simulink model "twoOctave"  (R2015a)
settings: Solver=ode45  StartTime=0.0  StopTime=480*640+7000  RelTol=1e-3
InitFcn:
  | %% DSPBuilder Start
  | alt_dspbuilder_update_model(bdroot)
  | %% DSPBuilder End
libraries: allblocks_alteradspbuilder2 x1298
(part 2 of 16)

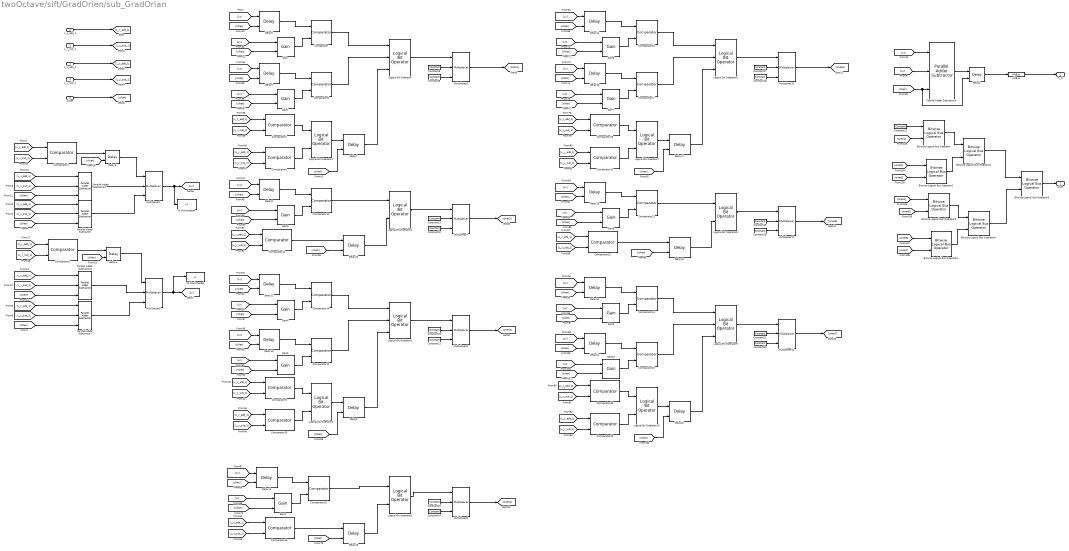
== system twoOctave/sift/GradOrien/sub_GradOrian ==
  L_y_add_1 : Inport
  L_x_add_1 : Inport  Port=2
  L_x_sub_1 : Inport  Port=3
  L_y_sub_1 : Inport  Port=4
  clken : Inport  Port=5
  AltBus : allblocks_alteradspbuilder2/AltBus  BusType=Unsigned Fractional  bwl=10  bwr=16  saturate=off  floatingPointInput=on  floatingPointOutput=on  logOutputs=off  logFile=C:\Users\ASUS\Desktop\final_sift_fpga\tb_twoOctave\twoOctave_sift_GradOrien_sub%5FGradOrian_AltBus.fixedpointlog
  Bitwise Logical Bus Operator{,1..6} (7 alike) : allblocks_alteradspbuilder2/Bitwise Logical Bus Operator  BusType=Unsigned Integer  bwl=3  bwr=0  LogicalOperator=OR  pipeline_display=0
  Comparator : allblocks_alteradspbuilder2/Comparator  direction=a >= b  pipeline_display=0  allowFloatingPointOverride=on  logOutputs=off  logFile=C:\Users\ASUS\Desktop\final_sift_fpga\tb_twoOctave\twoOctave_sift_GradOrien_sub%5FGradOrian_Comparator.fixedpointlog
  Comparator1 : allblocks_alteradspbuilder2/Comparator  direction=a > b  pipeline_display=0  allowFloatingPointOverride=on  logOutputs=off  logFile=C:\Users\ASUS\Desktop\final_sift_fpga\tb_twoOctave\twoOctave_sift_GradOrien_sub%5FGradOrian_Comparator1.fixedpointlog
  Comparator10 : allblocks_alteradspbuilder2/Comparator  direction=a >= b  pipeline_display=0  allowFloatingPointOverride=on  logOutputs=off  logFile=C:\Users\ASUS\Desktop\final_sift_fpga\tb_twoOctave\twoOctave_sift_GradOrien_sub%5FGradOrian_Comparator10.fixedpointlog
  Comparator11 : allblocks_alteradspbuilder2/Comparator  direction=a < b  pipeline_display=0  allowFloatingPointOverride=on  logOutputs=off  logFile=C:\Users\ASUS\Desktop\final_sift_fpga\tb_twoOctave\twoOctave_sift_GradOrien_sub%5FGradOrian_Comparator11.fixedpointlog
  Comparator12 : allblocks_alteradspbuilder2/Comparator  direction=a > b  pipeline_display=0  allowFloatingPointOverride=on  logOutputs=off  logFile=C:\Users\ASUS\Desktop\final_sift_fpga\tb_twoOctave\twoOctave_sift_GradOrien_sub%5FGradOrian_Comparator12.fixedpointlog
  Comparator13 : allblocks_alteradspbuilder2/Comparator  direction=a >= b  pipeline_display=0  allowFloatingPointOverride=on  logOutputs=off  logFile=C:\Users\ASUS\Desktop\final_sift_fpga\tb_twoOctave\twoOctave_sift_GradOrien_sub%5FGradOrian_Comparator13.fixedpointlog
  Comparator14 : allblocks_alteradspbuilder2/Comparator  direction=a >= b  pipeline_display=0  allowFloatingPointOverride=on  logOutputs=off  logFile=C:\Users\ASUS\Desktop\final_sift_fpga\tb_twoOctave\twoOctave_sift_GradOrien_sub%5FGradOrian_Comparator14.fixedpointlog
  Comparator15 : allblocks_alteradspbuilder2/Comparator  direction=a > b  pipeline_display=0  allowFloatingPointOverride=on  logOutputs=off  logFile=C:\Users\ASUS\Desktop\final_sift_fpga\tb_twoOctave\twoOctave_sift_GradOrien_sub%5FGradOrian_Comparator15.fixedpointlog
  Comparator16 : allblocks_alteradspbuilder2/Comparator  direction=a < b  pipeline_display=0  allowFloatingPointOverride=on  logOutputs=off  logFile=C:\Users\ASUS\Desktop\final_sift_fpga\tb_twoOctave\twoOctave_sift_GradOrien_sub%5FGradOrian_Comparator16.fixedpointlog
  Comparator17 : allblocks_alteradspbuilder2/Comparator  direction=a < b  pipeline_display=0  allowFloatingPointOverride=on  logOutputs=off  logFile=C:\Users\ASUS\Desktop\final_sift_fpga\tb_twoOctave\twoOctave_sift_GradOrien_sub%5FGradOrian_Comparator17.fixedpointlog
  Comparator18 : allblocks_alteradspbuilder2/Comparator  direction=a < b  pipeline_display=0  allowFloatingPointOverride=on  logOutputs=off  logFile=C:\Users\ASUS\Desktop\final_sift_fpga\tb_twoOctave\twoOctave_sift_GradOrien_sub%5FGradOrian_Comparator18.fixedpointlog
  Comparator19 : allblocks_alteradspbuilder2/Comparator  direction=a < b  pipeline_display=0  allowFloatingPointOverride=on  logOutputs=off  logFile=C:\Users\ASUS\Desktop\final_sift_fpga\tb_twoOctave\twoOctave_sift_GradOrien_sub%5FGradOrian_Comparator19.fixedpointlog
  Comparator2 : allblocks_alteradspbuilder2/Comparator  direction=a > b  pipeline_display=0  allowFloatingPointOverride=on  logOutputs=off  logFile=C:\Users\ASUS\Desktop\final_sift_fpga\tb_twoOctave\twoOctave_sift_GradOrien_sub%5FGradOrian_Comparator2.fixedpointlog
  Comparator20 : allblocks_alteradspbuilder2/Comparator  direction=a < b  pipeline_display=0  allowFloatingPointOverride=on  logOutputs=off  logFile=C:\Users\ASUS\Desktop\final_sift_fpga\tb_twoOctave\twoOctave_sift_GradOrien_sub%5FGradOrian_Comparator20.fixedpointlog
  Comparator21 : allblocks_alteradspbuilder2/Comparator  direction=a >= b  pipeline_display=0  allowFloatingPointOverride=on  logOutputs=off  logFile=C:\Users\ASUS\Desktop\final_sift_fpga\tb_twoOctave\twoOctave_sift_GradOrien_sub%5FGradOrian_Comparator21.fixedpointlog
  Comparator22 : allblocks_alteradspbuilder2/Comparator  direction=a < b  pipeline_display=0  allowFloatingPointOverride=on  logOutputs=off  logFile=C:\Users\ASUS\Desktop\final_sift_fpga\tb_twoOctave\twoOctave_sift_GradOrien_sub%5FGradOrian_Comparator22.fixedpointlog
  Comparator23 : allblocks_alteradspbuilder2/Comparator  direction=a < b  pipeline_display=0  allowFloatingPointOverride=on  logOutputs=off  logFile=C:\Users\ASUS\Desktop\final_sift_fpga\tb_twoOctave\twoOctave_sift_GradOrien_sub%5FGradOrian_Comparator23.fixedpointlog
  Comparator24 : allblocks_alteradspbuilder2/Comparator  direction=a >= b  pipeline_display=0  allowFloatingPointOverride=on  logOutputs=off  logFile=C:\Users\ASUS\Desktop\final_sift_fpga\tb_twoOctave\twoOctave_sift_GradOrien_sub%5FGradOrian_Comparator24.fixedpointlog
  Comparator25 : allblocks_alteradspbuilder2/Comparator  direction=a < b  pipeline_display=0  allowFloatingPointOverride=on  logOutputs=off  logFile=C:\Users\ASUS\Desktop\final_sift_fpga\tb_twoOctave\twoOctave_sift_GradOrien_sub%5FGradOrian_Comparator25.fixedpointlog
  Comparator26 : allblocks_alteradspbuilder2/Comparator  direction=a > b  pipeline_display=0  allowFloatingPointOverride=on  logOutputs=off  logFile=C:\Users\ASUS\Desktop\final_sift_fpga\tb_twoOctave\twoOctave_sift_GradOrien_sub%5FGradOrian_Comparator26.fixedpointlog
  Comparator6 : allblocks_alteradspbuilder2/Comparator  direction=a < b  pipeline_display=0  allowFloatingPointOverride=on  logOutputs=off  logFile=C:\Users\ASUS\Desktop\final_sift_fpga\tb_twoOctave\twoOctave_sift_GradOrien_sub%5FGradOrian_Comparator6.fixedpointlog
  Comparator7 : allblocks_alteradspbuilder2/Comparator  direction=a > b  pipeline_display=0  allowFloatingPointOverride=on  logOutputs=off  logFile=C:\Users\ASUS\Desktop\final_sift_fpga\tb_twoOctave\twoOctave_sift_GradOrien_sub%5FGradOrian_Comparator7.fixedpointlog
  Comparator8 : allblocks_alteradspbuilder2/Comparator  direction=a > b  pipeline_display=0  allowFloatingPointOverride=on  logOutputs=off  logFile=C:\Users\ASUS\Desktop\final_sift_fpga\tb_twoOctave\twoOctave_sift_GradOrien_sub%5FGradOrian_Comparator8.fixedpointlog
  Comparator9 : allblocks_alteradspbuilder2/Comparator  direction=a < b  pipeline_display=0  allowFloatingPointOverride=on  logOutputs=off  logFile=C:\Users\ASUS\Desktop\final_sift_fpga\tb_twoOctave\twoOctave_sift_GradOrien_sub%5FGradOrian_Comparator9.fixedpointlog
  Constant10 : allblocks_alteradspbuilder2/Constant  mask_cst=2  BusType=Unsigned Integer  bwl=3  bwr=0  roundMode=Truncate  satMode=Wrap  SpecifyClock=off  allowFloatingPointOverride=on  logOutputs=off  logFile=C:\Users\ASUS\Desktop\final_sift_fpga\tb_twoOctave\twoOctave_sift_GradOrien_sub%5FGradOrian_Constant10.fixedpointlog
  Constant11 : allblocks_alteradspbuilder2/Constant  mask_cst=0  BusType=Unsigned Integer  bwl=3  bwr=0  roundMode=Truncate  satMode=Wrap  SpecifyClock=off  allowFloatingPointOverride=on  logOutputs=off  logFile=C:\Users\ASUS\Desktop\final_sift_fpga\tb_twoOctave\twoOctave_sift_GradOrien_sub%5FGradOrian_Constant11.fixedpointlog
  Constant12 : allblocks_alteradspbuilder2/Constant  mask_cst=3  BusType=Unsigned Integer  bwl=3  bwr=0  roundMode=Truncate  satMode=Wrap  SpecifyClock=off  allowFloatingPointOverride=on  logOutputs=off  logFile=C:\Users\ASUS\Desktop\final_sift_fpga\tb_twoOctave\twoOctave_sift_GradOrien_sub%5FGradOrian_Constant12.fixedpointlog
  Constant13 : allblocks_alteradspbuilder2/Constant  mask_cst=0  BusType=Unsigned Integer  bwl=3  bwr=0  roundMode=Truncate  satMode=Wrap  SpecifyClock=off  allowFloatingPointOverride=on  logOutputs=off  logFile=C:\Users\ASUS\Desktop\final_sift_fpga\tb_twoOctave\twoOctave_sift_GradOrien_sub%5FGradOrian_Constant13.fixedpointlog
  Constant14 : allblocks_alteradspbuilder2/Constant  mask_cst=4  BusType=Unsigned Integer  bwl=3  bwr=0  roundMode=Truncate  satMode=Wrap  SpecifyClock=off  allowFloatingPointOverride=on  logOutputs=off  logFile=C:\Users\ASUS\Desktop\final_sift_fpga\tb_twoOctave\twoOctave_sift_GradOrien_sub%5FGradOrian_Constant14.fixedpointlog
  Constant15 : allblocks_alteradspbuilder2/Constant  mask_cst=0  BusType=Unsigned Integer  bwl=3  bwr=0  roundMode=Truncate  satMode=Wrap  SpecifyClock=off  allowFloatingPointOverride=on  logOutputs=off  logFile=C:\Users\ASUS\Desktop\final_sift_fpga\tb_twoOctave\twoOctave_sift_GradOrien_sub%5FGradOrian_Constant15.fixedpointlog
  Constant16 : allblocks_alteradspbuilder2/Constant  mask_cst=5  BusType=Unsigned Integer  bwl=3  bwr=0  roundMode=Truncate  satMode=Wrap  SpecifyClock=off  allowFloatingPointOverride=on  logOutputs=off  logFile=C:\Users\ASUS\Desktop\final_sift_fpga\tb_twoOctave\twoOctave_sift_GradOrien_sub%5FGradOrian_Constant16.fixedpointlog
  Constant17 : allblocks_alteradspbuilder2/Constant  mask_cst=0  BusType=Unsigned Integer  bwl=3  bwr=0  roundMode=Truncate  satMode=Wrap  SpecifyClock=off  allowFloatingPointOverride=on  logOutputs=off  logFile=C:\Users\ASUS\Desktop\final_sift_fpga\tb_twoOctave\twoOctave_sift_GradOrien_sub%5FGradOrian_Constant17.fixedpointlog
  Constant18 : allblocks_alteradspbuilder2/Constant  mask_cst=6  BusType=Unsigned Integer  bwl=3  bwr=0  roundMode=Truncate  satMode=Wrap  SpecifyClock=off  allowFloatingPointOverride=on  logOutputs=off  logFile=C:\Users\ASUS\Desktop\final_sift_fpga\tb_twoOctave\twoOctave_sift_GradOrien_sub%5FGradOrian_Constant18.fixedpointlog
  Constant19 : allblocks_alteradspbuilder2/Constant  mask_cst=0  BusType=Unsigned Integer  bwl=3  bwr=0  roundMode=Truncate  satMode=Wrap  SpecifyClock=off  allowFloatingPointOverride=on  logOutputs=off  logFile=C:\Users\ASUS\Desktop\final_sift_fpga\tb_twoOctave\twoOctave_sift_GradOrien_sub%5FGradOrian_Constant19.fixedpointlog
  Constant20 : allblocks_alteradspbuilder2/Constant  mask_cst=7  BusType=Unsigned Integer  bwl=3  bwr=0  roundMode=Truncate  satMode=Wrap  SpecifyClock=off  allowFloatingPointOverride=on  logOutputs=off  logFile=C:\Users\ASUS\Desktop\final_sift_fpga\tb_twoOctave\twoOctave_sift_GradOrien_sub%5FGradOrian_Constant20.fixedpointlog
  Constant21 : allblocks_alteradspbuilder2/Constant  mask_cst=0  BusType=Unsigned Integer  bwl=3  bwr=0  roundMode=Truncate  satMode=Wrap  SpecifyClock=off  allowFloatingPointOverride=on  logOutputs=off  logFile=C:\Users\ASUS\Desktop\final_sift_fpga\tb_twoOctave\twoOctave_sift_GradOrien_sub%5FGradOrian_Constant21.fixedpointlog
  Constant22 : allblocks_alteradspbuilder2/Constant  mask_cst=0  BusType=Unsigned Integer  bwl=3  bwr=0  roundMode=Truncate  satMode=Wrap  SpecifyClock=off  allowFloatingPointOverride=on  logOutputs=off  logFile=C:\Users\ASUS\Desktop\final_sift_fpga\tb_twoOctave\twoOctave_sift_GradOrien_sub%5FGradOrian_Constant22.fixedpointlog
  Constant8 : allblocks_alteradspbuilder2/Constant  mask_cst=1  BusType=Unsigned Integer  bwl=3  bwr=0  roundMode=Truncate  satMode=Wrap  SpecifyClock=off  allowFloatingPointOverride=on  logOutputs=off  logFile=C:\Users\ASUS\Desktop\final_sift_fpga\tb_twoOctave\twoOctave_sift_GradOrien_sub%5FGradOrian_Constant8.fixedpointlog
  Constant9 : allblocks_alteradspbuilder2/Constant  mask_cst=0  BusType=Unsigned Integer  bwl=3  bwr=0  roundMode=Truncate  satMode=Wrap  SpecifyClock=off  allowFloatingPointOverride=on  logOutputs=off  logFile=C:\Users\ASUS\Desktop\final_sift_fpga\tb_twoOctave\twoOctave_sift_GradOrien_sub%5FGradOrian_Constant9.fixedpointlog
  Delay1 : allblocks_alteradspbuilder2/Delay  pipeline=15  pipeline_display=15  ClockPhase=1  use_ena=on  use_sclr=off  allowFloatingPointOverride=on  logOutputs=off  logFile=C:\Users\ASUS\Desktop\final_sift_fpga\tb_twoOctave\twoOctave_sift_GradOrien_sub%5FGradOrian_Delay1.fixedpointlog  use_init=off  reset_value=1
  Delay10 : allblocks_alteradspbuilder2/Delay  pipeline=17  pipeline_display=17  ClockPhase=1  use_ena=on  use_sclr=off  allowFloatingPointOverride=on  logOutputs=off  logFile=C:\Users\ASUS\Desktop\final_sift_fpga\tb_twoOctave\twoOctave_sift_GradOrien_sub%5FGradOrian_Delay10.fixedpointlog  use_init=off  reset_value=1
  Delay11 : allblocks_alteradspbuilder2/Delay  pipeline=16  pipeline_display=16  ClockPhase=1  use_ena=on  use_sclr=off  allowFloatingPointOverride=on  logOutputs=off  logFile=C:\Users\ASUS\Desktop\final_sift_fpga\tb_twoOctave\twoOctave_sift_GradOrien_sub%5FGradOrian_Delay11.fixedpointlog  use_init=off  reset_value=1
  Delay12 : allblocks_alteradspbuilder2/Delay  pipeline=16  pipeline_display=16  ClockPhase=1  use_ena=on  use_sclr=off  allowFloatingPointOverride=on  logOutputs=off  logFile=C:\Users\ASUS\Desktop\final_sift_fpga\tb_twoOctave\twoOctave_sift_GradOrien_sub%5FGradOrian_Delay12.fixedpointlog  use_init=off  reset_value=1
  Delay13 : allblocks_alteradspbuilder2/Delay  pipeline=16  pipeline_display=16  ClockPhase=1  use_ena=on  use_sclr=off  allowFloatingPointOverride=on  logOutputs=off  logFile=C:\Users\ASUS\Desktop\final_sift_fpga\tb_twoOctave\twoOctave_sift_GradOrien_sub%5FGradOrian_Delay13.fixedpointlog  use_init=off  reset_value=1
  Delay14 : allblocks_alteradspbuilder2/Delay  pipeline=16  pipeline_display=16  ClockPhase=1  use_ena=on  use_sclr=off  allowFloatingPointOverride=on  logOutputs=off  logFile=C:\Users\ASUS\Desktop\final_sift_fpga\tb_twoOctave\twoOctave_sift_GradOrien_sub%5FGradOrian_Delay14.fixedpointlog  use_init=off  reset_value=1
  Delay15 : allblocks_alteradspbuilder2/Delay  pipeline=17  pipeline_display=17  ClockPhase=1  use_ena=on  use_sclr=off  allowFloatingPointOverride=on  logOutputs=off  logFile=C:\Users\ASUS\Desktop\final_sift_fpga\tb_twoOctave\twoOctave_sift_GradOrien_sub%5FGradOrian_Delay15.fixedpointlog  use_init=off  reset_value=1
  Delay16 : allblocks_alteradspbuilder2/Delay  pipeline=16  pipeline_display=16  ClockPhase=1  use_ena=on  use_sclr=off  allowFloatingPointOverride=on  logOutputs=off  logFile=C:\Users\ASUS\Desktop\final_sift_fpga\tb_twoOctave\twoOctave_sift_GradOrien_sub%5FGradOrian_Delay16.fixedpointlog  use_init=off  reset_value=1
  Delay17 : allblocks_alteradspbuilder2/Delay  pipeline=17  pipeline_display=17  ClockPhase=1  use_ena=on  use_sclr=off  allowFloatingPointOverride=on  logOutputs=off  logFile=C:\Users\ASUS\Desktop\final_sift_fpga\tb_twoOctave\twoOctave_sift_GradOrien_sub%5FGradOrian_Delay17.fixedpointlog  use_init=off  reset_value=1
  Delay18 : allblocks_alteradspbuilder2/Delay  pipeline=17  pipeline_display=17  ClockPhase=1  use_ena=on  use_sclr=off  allowFloatingPointOverride=on  logOutputs=off  logFile=C:\Users\ASUS\Desktop\final_sift_fpga\tb_twoOctave\twoOctave_sift_GradOrien_sub%5FGradOrian_Delay18.fixedpointlog  use_init=off  reset_value=1
  Delay19 : allblocks_alteradspbuilder2/Delay  pipeline=16  pipeline_display=16  ClockPhase=1  use_ena=on  use_sclr=off  allowFloatingPointOverride=on  logOutputs=off  logFile=C:\Users\ASUS\Desktop\final_sift_fpga\tb_twoOctave\twoOctave_sift_GradOrien_sub%5FGradOrian_Delay19.fixedpointlog  use_init=off  reset_value=1
  Delay20 : allblocks_alteradspbuilder2/Delay  pipeline=16  pipeline_display=16  ClockPhase=1  use_ena=on  use_sclr=off  allowFloatingPointOverride=on  logOutputs=off  logFile=C:\Users\ASUS\Desktop\final_sift_fpga\tb_twoOctave\twoOctave_sift_GradOrien_sub%5FGradOrian_Delay20.fixedpointlog  use_init=off  reset_value=1
  Delay21 : allblocks_alteradspbuilder2/Delay  pipeline=16  pipeline_display=16  ClockPhase=1  use_ena=on  use_sclr=off  allowFloatingPointOverride=on  logOutputs=off  logFile=C:\Users\ASUS\Desktop\final_sift_fpga\tb_twoOctave\twoOctave_sift_GradOrien_sub%5FGradOrian_Delay21.fixedpointlog  use_init=off  reset_value=1
  Delay22 : allblocks_alteradspbuilder2/Delay  pipeline=17  pipeline_display=17  ClockPhase=1  use_ena=on  use_sclr=off  allowFloatingPointOverride=on  logOutputs=off  logFile=C:\Users\ASUS\Desktop\final_sift_fpga\tb_twoOctave\twoOctave_sift_GradOrien_sub%5FGradOrian_Delay22.fixedpointlog  use_init=off  reset_value=1
  Delay3 : allblocks_alteradspbuilder2/Delay  pipeline=1  pipeline_display=1  ClockPhase=1  use_ena=on  use_sclr=off  allowFloatingPointOverride=on  logOutputs=off  logFile=C:\Users\ASUS\Desktop\final_sift_fpga\tb_twoOctave\twoOctave_sift_GradOrien_sub%5FGradOrian_Delay3.fixedpointlog  use_init=off  reset_value=1
  Delay4 : allblocks_alteradspbuilder2/Delay  pipeline=1  pipeline_display=1  ClockPhase=1  use_ena=on  use_sclr=off  allowFloatingPointOverride=on  logOutputs=off  logFile=C:\Users\ASUS\Desktop\final_sift_fpga\tb_twoOctave\twoOctave_sift_GradOrien_sub%5FGradOrian_Delay4.fixedpointlog  use_init=off  reset_value=1
  Delay5 : allblocks_alteradspbuilder2/Delay  pipeline=16  pipeline_display=16  ClockPhase=1  use_ena=on  use_sclr=off  allowFloatingPointOverride=on  logOutputs=off  logFile=C:\Users\ASUS\Desktop\final_sift_fpga\tb_twoOctave\twoOctave_sift_GradOrien_sub%5FGradOrian_Delay5.fixedpointlog  use_init=off  reset_value=1
  Delay6 : allblocks_alteradspbuilder2/Delay  pipeline=16  pipeline_display=16  ClockPhase=1  use_ena=on  use_sclr=off  allowFloatingPointOverride=on  logOutputs=off  logFile=C:\Users\ASUS\Desktop\final_sift_fpga\tb_twoOctave\twoOctave_sift_GradOrien_sub%5FGradOrian_Delay6.fixedpointlog  use_init=off  reset_value=1
  Delay7 : allblocks_alteradspbuilder2/Delay  pipeline=17  pipeline_display=17  ClockPhase=1  use_ena=on  use_sclr=off  allowFloatingPointOverride=on  logOutputs=off  logFile=C:\Users\ASUS\Desktop\final_sift_fpga\tb_twoOctave\twoOctave_sift_GradOrien_sub%5FGradOrian_Delay7.fixedpointlog  use_init=off  reset_value=1
  Delay8 : allblocks_alteradspbuilder2/Delay  pipeline=17  pipeline_display=17  ClockPhase=1  use_ena=on  use_sclr=off  allowFloatingPointOverride=on  logOutputs=off  logFile=C:\Users\ASUS\Desktop\final_sift_fpga\tb_twoOctave\twoOctave_sift_GradOrien_sub%5FGradOrian_Delay8.fixedpointlog  use_init=off  reset_value=1
  Delay9 : allblocks_alteradspbuilder2/Delay  pipeline=16  pipeline_display=16  ClockPhase=1  use_ena=on  use_sclr=off  allowFloatingPointOverride=on  logOutputs=off  logFile=C:\Users\ASUS\Desktop\final_sift_fpga\tb_twoOctave\twoOctave_sift_GradOrien_sub%5FGradOrian_Delay9.fixedpointlog  use_init=off  reset_value=1
  Gain : allblocks_alteradspbuilder2/Gain  vgain=0.414  BusType=Unsigned Fractional  bwl=8  bwr=16  pipeline=16  pipeline_display=16  allowFloatingPointOverride=on  logOutputs=off  logFile=C:\Users\ASUS\Desktop\final_sift_fpga\tb_twoOctave\twoOctave_sift_GradOrien_sub%5FGradOrian_Gain.fixedpointlog  use_ena=on  use_aclr=off  lpm=off  MaskValue=1
  Gain1 : allblocks_alteradspbuilder2/Gain  vgain=2.414  BusType=Unsigned Fractional  bwl=8  bwr=16  pipeline=16  pipeline_display=16  allowFloatingPointOverride=on  logOutputs=off  logFile=C:\Users\ASUS\Desktop\final_sift_fpga\tb_twoOctave\twoOctave_sift_GradOrien_sub%5FGradOrian_Gain1.fixedpointlog  use_ena=on  use_aclr=off  lpm=off  MaskValue=1
  Gain10 : allblocks_alteradspbuilder2/Gain  vgain=2.414  BusType=Unsigned Fractional  bwl=8  bwr=16  pipeline=16  pipeline_display=16  allowFloatingPointOverride=on  logOutputs=off  logFile=C:\Users\ASUS\Desktop\final_sift_fpga\tb_twoOctave\twoOctave_sift_GradOrien_sub%5FGradOrian_Gain10.fixedpointlog  use_ena=on  use_aclr=off  lpm=off  MaskValue=1
  Gain2 : allblocks_alteradspbuilder2/Gain  vgain=0.414  BusType=Unsigned Fractional  bwl=8  bwr=16  pipeline=16  pipeline_display=16  allowFloatingPointOverride=on  logOutputs=off  logFile=C:\Users\ASUS\Desktop\final_sift_fpga\tb_twoOctave\twoOctave_sift_GradOrien_sub%5FGradOrian_Gain2.fixedpointlog  use_ena=on  use_aclr=off  lpm=off  MaskValue=1
  Gain3 : allblocks_alteradspbuilder2/Gain  vgain=2.414  BusType=Unsigned Fractional  bwl=8  bwr=16  pipeline=16  pipeline_display=16  allowFloatingPointOverride=on  logOutputs=off  logFile=C:\Users\ASUS\Desktop\final_sift_fpga\tb_twoOctave\twoOctave_sift_GradOrien_sub%5FGradOrian_Gain3.fixedpointlog  use_ena=on  use_aclr=off  lpm=off  MaskValue=1
  Gain4 : allblocks_alteradspbuilder2/Gain  vgain=0.414  BusType=Unsigned Fractional  bwl=8  bwr=16  pipeline=16  pipeline_display=16  allowFloatingPointOverride=on  logOutputs=off  logFile=C:\Users\ASUS\Desktop\final_sift_fpga\tb_twoOctave\twoOctave_sift_GradOrien_sub%5FGradOrian_Gain4.fixedpointlog  use_ena=on  use_aclr=off  lpm=off  MaskValue=1
  Gain5 : allblocks_alteradspbuilder2/Gain  vgain=2.414  BusType=Unsigned Fractional  bwl=8  bwr=16  pipeline=16  pipeline_display=16  allowFloatingPointOverride=on  logOutputs=off  logFile=C:\Users\ASUS\Desktop\final_sift_fpga\tb_twoOctave\twoOctave_sift_GradOrien_sub%5FGradOrian_Gain5.fixedpointlog  use_ena=on  use_aclr=off  lpm=off  MaskValue=1
  Gain6 : allblocks_alteradspbuilder2/Gain  vgain=0.414  BusType=Unsigned Fractional  bwl=8  bwr=16  pipeline=16  pipeline_display=16  allowFloatingPointOverride=on  logOutputs=off  logFile=C:\Users\ASUS\Desktop\final_sift_fpga\tb_twoOctave\twoOctave_sift_GradOrien_sub%5FGradOrian_Gain6.fixedpointlog  use_ena=on  use_aclr=off  lpm=off  MaskValue=1
  Gain7 : allblocks_alteradspbuilder2/Gain  vgain=2.414  BusType=Unsigned Fractional  bwl=8  bwr=16  pipeline=16  pipeline_display=16  allowFloatingPointOverride=on  logOutputs=off  logFile=C:\Users\ASUS\Desktop\final_sift_fpga\tb_twoOctave\twoOctave_sift_GradOrien_sub%5FGradOrian_Gain7.fixedpointlog  use_ena=on  use_aclr=off  lpm=off  MaskValue=1
  Gain8 : allblocks_alteradspbuilder2/Gain  vgain=2.414  BusType=Unsigned Fractional  bwl=8  bwr=16  pipeline=16  pipeline_display=16  allowFloatingPointOverride=on  logOutputs=off  logFile=C:\Users\ASUS\Desktop\final_sift_fpga\tb_twoOctave\twoOctave_sift_GradOrien_sub%5FGradOrian_Gain8.fixedpointlog  use_ena=on  use_aclr=off  lpm=off  MaskValue=1
  Gain9 : allblocks_alteradspbuilder2/Gain  vgain=0.414  BusType=Unsigned Fractional  bwl=8  bwr=16  pipeline=16  pipeline_display=16  allowFloatingPointOverride=on  logOutputs=off  logFile=C:\Users\ASUS\Desktop\final_sift_fpga\tb_twoOctave\twoOctave_sift_GradOrien_sub%5FGradOrian_Gain9.fixedpointlog  use_ena=on  use_aclr=off  lpm=off  MaskValue=1
  Logical Bit Operator{,3,6,9} (4 alike) : allblocks_alteradspbuilder2/Logical Bit Operator  LogicalOperator=AND  user_inputs=3  pipeline_display=0
  Logical Bit Operator{1..2,4..5,7..8,10} (7 alike) : allblocks_alteradspbuilder2/Logical Bit Operator  LogicalOperator=AND  user_inputs=2  pipeline_display=0
  Multiplexer1 : allblocks_alteradspbuilder2/Multiplexer  numInputs=2  pipeline=0  oneHot=off  pipeline_display=0  use_ena=off  use_aclr=off  allowFloatingPointOverride=on  logOutputs=off  logFile=C:\Users\ASUS\Desktop\final_sift_fpga\tb_twoOctave\twoOctave_sift_GradOrien_sub%5FGradOrian_Multiplexer1.fixedpointlog
  Multiplexer10 : allblocks_alteradspbuilder2/Multiplexer  numInputs=2  pipeline=0  oneHot=off  pipeline_display=0  use_ena=off  use_aclr=off  allowFloatingPointOverride=on  logOutputs=off  logFile=C:\Users\ASUS\Desktop\final_sift_fpga\tb_twoOctave\twoOctave_sift_GradOrien_sub%5FGradOrian_Multiplexer10.fixedpointlog
  Multiplexer11 : allblocks_alteradspbuilder2/Multiplexer  numInputs=2  pipeline=0  oneHot=off  pipeline_display=0  use_ena=off  use_aclr=off  allowFloatingPointOverride=on  logOutputs=off  logFile=C:\Users\ASUS\Desktop\final_sift_fpga\tb_twoOctave\twoOctave_sift_GradOrien_sub%5FGradOrian_Multiplexer11.fixedpointlog
  Multiplexer12 : allblocks_alteradspbuilder2/Multiplexer  numInputs=2  pipeline=0  oneHot=off  pipeline_display=0  use_ena=off  use_aclr=off  allowFloatingPointOverride=on  logOutputs=off  logFile=C:\Users\ASUS\Desktop\final_sift_fpga\tb_twoOctave\twoOctave_sift_GradOrien_sub%5FGradOrian_Multiplexer12.fixedpointlog
  Multiplexer5 : allblocks_alteradspbuilder2/Multiplexer  numInputs=2  pipeline=0  oneHot=off  pipeline_display=0  use_ena=off  use_aclr=off  allowFloatingPointOverride=on  logOutputs=off  logFile=C:\Users\ASUS\Desktop\final_sift_fpga\tb_twoOctave\twoOctave_sift_GradOrien_sub%5FGradOrian_Multiplexer5.fixedpointlog
  Multiplexer6 : allblocks_alteradspbuilder2/Multiplexer  numInputs=2  pipeline=0  oneHot=off  pipeline_display=0  use_ena=off  use_aclr=off  allowFloatingPointOverride=on  logOutputs=off  logFile=C:\Users\ASUS\Desktop\final_sift_fpga\tb_twoOctave\twoOctave_sift_GradOrien_sub%5FGradOrian_Multiplexer6.fixedpointlog
  Multiplexer7 : allblocks_alteradspbuilder2/Multiplexer  numInputs=2  pipeline=0  oneHot=off  pipeline_display=0  use_ena=off  use_aclr=off  allowFloatingPointOverride=on  logOutputs=off  logFile=C:\Users\ASUS\Desktop\final_sift_fpga\tb_twoOctave\twoOctave_sift_GradOrien_sub%5FGradOrian_Multiplexer7.fixedpointlog
  Multiplexer8 : allblocks_alteradspbuilder2/Multiplexer  numInputs=2  pipeline=0  oneHot=off  pipeline_display=0  use_ena=off  use_aclr=off  allowFloatingPointOverride=on  logOutputs=off  logFile=C:\Users\ASUS\Desktop\final_sift_fpga\tb_twoOctave\twoOctave_sift_GradOrien_sub%5FGradOrian_Multiplexer8.fixedpointlog
  Multiplexer9 : allblocks_alteradspbuilder2/Multiplexer  numInputs=2  pipeline=0  oneHot=off  pipeline_display=0  use_ena=off  use_aclr=off  allowFloatingPointOverride=on  logOutputs=off  logFile=C:\Users\ASUS\Desktop\final_sift_fpga\tb_twoOctave\twoOctave_sift_GradOrien_sub%5FGradOrian_Multiplexer9.fixedpointlog
  Parallel Adder Subtractor : allblocks_alteradspbuilder2/Parallel Adder Subtractor  number_of_inputs=2  direction=+-  use_pipeline=on  pipeline_display=1  phase_selection=1  use_ena=on  use_aclr=off  allowFloatingPointOverride=on  logOutputs=off  logFile=C:\Users\ASUS\Desktop\final_sift_fpga\tb_twoOctave\twoOctave_sift_GradOrien_sub%5FGradOrian_Parallel+Adder+Subtractor.fixedpointlog
  Parallel Adder Subtractor1 : allblocks_alteradspbuilder2/Parallel Adder Subtractor  number_of_inputs=2  direction=+-  use_pipeline=on  pipeline_display=1  phase_selection=1  use_ena=on  use_aclr=off  allowFloatingPointOverride=on  logOutputs=off  logFile=C:\Users\ASUS\Desktop\final_sift_fpga\tb_twoOctave\twoOctave_sift_GradOrien_sub%5FGradOrian_Parallel+Adder+Subtractor1.fixedpointlog
  Parallel Adder Subtractor2 : allblocks_alteradspbuilder2/Parallel Adder Subtractor  number_of_inputs=2  direction=-+  use_pipeline=on  pipeline_display=1  phase_selection=1  use_ena=on  use_aclr=off  allowFloatingPointOverride=on  logOutputs=off  logFile=C:\Users\ASUS\Desktop\final_sift_fpga\tb_twoOctave\twoOctave_sift_GradOrien_sub%5FGradOrian_Parallel+Adder+Subtractor2.fixedpointlog
  Parallel Adder Subtractor3 : allblocks_alteradspbuilder2/Parallel Adder Subtractor  number_of_inputs=2  direction=-+  use_pipeline=on  pipeline_display=1  phase_selection=1  use_ena=on  use_aclr=off  allowFloatingPointOverride=on  logOutputs=off  logFile=C:\Users\ASUS\Desktop\final_sift_fpga\tb_twoOctave\twoOctave_sift_GradOrien_sub%5FGradOrian_Parallel+Adder+Subtractor3.fixedpointlog
  Parallel Adder Subtractor5 : allblocks_alteradspbuilder2/Parallel Adder Subtractor  number_of_inputs=2  direction=++  use_pipeline=on  pipeline_display=1  phase_selection=1  use_ena=on  use_aclr=off  allowFloatingPointOverride=on  logOutputs=off  logFile=C:\Users\ASUS\Desktop\final_sift_fpga\tb_twoOctave\twoOctave_sift_GradOrien_sub%5FGradOrian_Parallel+Adder+Subtractor5.fixedpointlog
  To Workspace4 : ToWorkspace  VariableName=Lx  SaveFormat=Timeseries  SampleTime=-1
  To Workspace6 : ToWorkspace  VariableName=Ly  SaveFormat=Timeseries  SampleTime=-1
  orien : Outport
  m_xy : Outport  Port=2
  wires:
  [clken] -> Delay1/2, Parallel Adder Subtractor5/3
  L_x_add_1/1 -> [L_x_add_1]
  AltBus/1 -> m_xy/1
  clken/1 -> [clken]
  Parallel Adder Subtractor5/1 -> Delay1/1
  Parallel Adder Subtractor2/1 -> Multiplexer1/2
  [clken] -> Parallel Adder Subtractor2/3
  [L_y_add_1] -> Parallel Adder Subtractor3/1
  Parallel Adder Subtractor3/1 -> Multiplexer5/2
  [L_y_sub_1] -> Parallel Adder Subtractor3/2
  [L_x_sub_1] -> Parallel Adder Subtractor2/2
  [clken] -> Parallel Adder Subtractor3/3
  [L_x_add_1] -> Parallel Adder Subtractor2/1
  [L_x_sub_1] -> Parallel Adder Subtractor/2
  [L_y_sub_1] -> Parallel Adder Subtractor1/2
  [L_y_add_1] -> Parallel Adder Subtractor1/1
  [clken] -> Parallel Adder Subtractor/3
  Parallel Adder Subtractor/1 -> Multiplexer1/3
  Parallel Adder Subtractor1/1 -> Multiplexer5/3
  [clken] -> Parallel Adder Subtractor1/3
  [L_x_add_1] -> Parallel Adder Subtractor/1
  Comparator1/1 -> Delay3/1
  [L_x_sub_1] -> Comparator1/2
  [L_x_add_1] -> Comparator1/1
  [clken] -> Delay3/2
  Delay3/1 -> Multiplexer1/1
  Multiplexer1/1 -> To Workspace4/1, [Lx]
  [L_y_sub_1] -> Comparator2/2
  [L_y_add_1] -> Comparator2/1
  [clken] -> Delay4/2
  Comparator2/1 -> Delay4/1
  Delay4/1 -> Multiplexer5/1
  [Ly] -> Delay5/1
  [clken] -> Delay5/2
  [Lx] -> Gain/1
  [clken] -> Gain/2
  Delay5/1 -> Comparator/1
  Gain/1 -> Comparator/2
  Comparator/1 -> Logical Bit Operator/1
  [Ly] -> Delay6/1
  [clken] -> Delay6/2
  [Lx] -> Gain1/1
  [clken] -> Gain1/2
  Delay6/1 -> Comparator6/1
  Gain1/1 -> Comparator6/2
  Comparator6/1 -> Logical Bit Operator/2
  Logical Bit Operator/1 -> Multiplexer6/1
  [L_y_sub_1] -> Comparator8/2
  [L_x_sub_1] -> Comparator7/2
  [L_y_add_1] -> Comparator8/1
  [L_x_add_1] -> Comparator7/1
  Comparator7/1 -> Logical Bit Operator1/1
  Comparator8/1 -> Logical Bit Operator1/2
  Logical Bit Operator1/1 -> Delay7/1
  [clken] -> Delay7/2
  Delay7/1 -> Logical Bit Operator/3
  Constant8/1 -> Multiplexer6/3
  Constant9/1 -> Multiplexer6/2
  Multiplexer6/1 -> [orien1]
  [Ly] -> Delay9/1
  [clken] -> Delay9/2
  [Lx] -> Gain3/1
  [clken] -> Gain3/2
  Delay9/1 -> Comparator10/1
  Gain3/1 -> Comparator10/2
  Comparator10/1 -> Logical Bit Operator2/1
  Logical Bit Operator2/1 -> Multiplexer7/1
  [L_y_sub_1] -> Comparator12/2
  [L_y_add_1] -> Comparator12/1
  Comparator12/1 -> Delay10/1
  [clken] -> Delay10/2
  Delay10/1 -> Logical Bit Operator2/2
  Constant10/1 -> Multiplexer7/3
  Constant11/1 -> Multiplexer7/2
  Multiplexer7/1 -> [orien2]
  [Ly] -> Delay12/1
  [clken] -> Delay12/2
  [Lx] -> Gain4/1
  [clken] -> Gain4/2
  Delay12/1 -> Comparator14/1
  Gain4/1 -> Comparator14/2
  Comparator14/1 -> Logical Bit Operator3/1
  [Ly] -> Delay13/1
  [clken] -> Delay13/2
  [Lx] -> Gain5/1
  [clken] -> Gain5/2
  Delay13/1 -> Comparator11/1
  Gain5/1 -> Comparator11/2
  Comparator11/1 -> Logical Bit Operator3/2
  Logical Bit Operator3/1 -> Multiplexer8/1
  Constant12/1 -> Multiplexer8/3
  Constant13/1 -> Multiplexer8/2
  Multiplexer8/1 -> [orien3]
  [L_y_sub_1] -> Comparator15/2
  [L_x_sub_1] -> Comparator9/2
  [L_y_add_1] -> Comparator15/1
  [L_x_add_1] -> Comparator9/1
  Comparator9/1 -> Logical Bit Operator4/1
  Comparator15/1 -> Logical Bit Operator4/2
  Logical Bit Operator4/1 -> Delay8/1
  [clken] -> Delay8/2
  Delay8/1 -> Logical Bit Operator3/3
  [Ly] -> Delay11/1
  [clken] -> Delay11/2
  [Lx] -> Gain2/1
  [clken] -> Gain2/2
  Delay11/1 -> Comparator16/1
  Gain2/1 -> Comparator16/2
  Comparator16/1 -> Logical Bit Operator5/1
  Logical Bit Operator5/1 -> Multiplexer9/1
  Constant14/1 -> Multiplexer9/3
  Constant15/1 -> Multiplexer9/2
  Multiplexer9/1 -> [orien4]
  [L_x_sub_1] -> Comparator18/2
  [L_x_add_1] -> Comparator18/1
  Comparator18/1 -> Delay15/1
  [clken] -> Delay15/2
  Delay15/1 -> Logical Bit Operator5/2
  [Ly] -> Delay14/1
  [clken] -> Delay14/2
  [Lx] -> Gain6/1
  [clken] -> Gain6/2
  Delay14/1 -> Comparator13/1
  Gain6/1 -> Comparator13/2
  Comparator13/1 -> Logical Bit Operator6/1
  [Ly] -> Delay16/1
  [clken] -> Delay16/2
  [Lx] -> Gain7/1
  [clken] -> Gain7/2
  Delay16/1 -> Comparator17/1
  Gain7/1 -> Comparator17/2
  Comparator17/1 -> Logical Bit Operator6/2
  Logical Bit Operator6/1 -> Multiplexer10/1
  [L_y_sub_1] -> Comparator20/2
  [L_x_sub_1] -> Comparator19/2
  [L_y_add_1] -> Comparator20/1
  [L_x_add_1] -> Comparator19/1
  Comparator19/1 -> Logical Bit Operator7/1
  Comparator20/1 -> Logical Bit Operator7/2
  Logical Bit Operator7/1 -> Delay17/1
  [clken] -> Delay17/2
  Delay17/1 -> Logical Bit Operator6/3
  Constant16/1 -> Multiplexer10/3
  Constant17/1 -> Multiplexer10/2
  Multiplexer10/1 -> [orien5]
  [clken] -> Delay19/2
  [Lx] -> Gain8/1
  [clken] -> Gain8/2
  Delay19/1 -> Comparator21/1
  Gain8/1 -> Comparator21/2
  Comparator21/1 -> Logical Bit Operator8/1
  Logical Bit Operator8/1 -> Multiplexer11/1
  [L_y_sub_1] -> Comparator22/2
  [L_y_add_1] -> Comparator22/1
  Comparator22/1 -> Delay18/1
  Delay18/1 -> Logical Bit Operator8/2
  Constant18/1 -> Multiplexer11/3
  Constant19/1 -> Multiplexer11/2
  Multiplexer11/1 -> [orien6]
  [Ly] -> Delay19/1
  [Ly] -> Delay20/1
  [clken] -> Delay20/2
  [Lx] -> Gain9/1
  [clken] -> Gain9/2
  Delay20/1 -> Comparator24/1
  Gain9/1 -> Comparator24/2
  Comparator24/1 -> Logical Bit Operator9/1
  [Ly] -> Delay21/1
  [clken] -> Delay21/2
  [Lx] -> Gain10/1
  [clken] -> Gain10/2
  Delay21/1 -> Comparator23/1
  Gain10/1 -> Comparator23/2
  Comparator23/1 -> Logical Bit Operator9/2
  Logical Bit Operator9/1 -> Multiplexer12/1
  Constant20/1 -> Multiplexer12/3
  Constant21/1 -> Multiplexer12/2
  Multiplexer12/1 -> [orien7]
  [L_y_sub_1] -> Comparator25/2
  [L_x_sub_1] -> Comparator26/2
  [L_y_add_1] -> Comparator25/1
  [L_x_add_1] -> Comparator26/1
  Comparator26/1 -> Logical Bit Operator10/1
  Comparator25/1 -> Logical Bit Operator10/2
  Logical Bit Operator10/1 -> Delay22/1
  [clken] -> Delay22/2
  Delay22/1 -> Logical Bit Operator9/3
  [orien1] -> Bitwise Logical Bus Operator/2
  Constant22/1 -> Bitwise Logical Bus Operator/1
  [orien3] -> Bitwise Logical Bus Operator1/2
  [orien2] -> Bitwise Logical Bus Operator1/1
  Bitwise Logical Bus Operator/1 -> Bitwise Logical Bus Operator2/1
  Bitwise Logical Bus Operator1/1 -> Bitwise Logical Bus Operator2/2
  [orien5] -> Bitwise Logical Bus Operator3/2
  [orien4] -> Bitwise Logical Bus Operator3/1
  [orien7] -> Bitwise Logical Bus Operator4/2
  [orien6] -> Bitwise Logical Bus Operator4/1
  Bitwise Logical Bus Operator3/1 -> Bitwise Logical Bus Operator5/1
  Bitwise Logical Bus Operator4/1 -> Bitwise Logical Bus Operator5/2
  Bitwise Logical Bus Operator2/1 -> Bitwise Logical Bus Operator6/1
  Bitwise Logical Bus Operator5/1 -> Bitwise Logical Bus Operator6/2
  Bitwise Logical Bus Operator6/1 -> orien/1
  [Ly] -> Parallel Adder Subtractor5/2
  [Lx] -> Parallel Adder Subtractor5/1
  Delay1/1 -> AltBus/1
  [clken] -> Delay18/2
  L_x_sub_1/1 -> [L_x_sub_1]
  L_y_add_1/1 -> [L_y_add_1]
  L_y_sub_1/1 -> [L_y_sub_1]
  Multiplexer5/1 -> To Workspace6/1, [Ly]

== system twoOctave/sift/SIFT_detector/Octave0 ==
  data_in : Inport
  valid_in : Inport  Port=2
  detect_keypoint : Subsystem
  dog_space : Subsystem
  scale_space : Subsystem
  is_Keypoint : Outport
  scale2 : Outport  Port=2
  wires:
  scale_space/3(scale2) -> scale2/1, dog_space/3(scale2_in)
  scale_space/1(scale4) -> dog_space/1(scale4_in)
  scale_space/4(scale1) -> dog_space/4(scale1_in)
  detect_keypoint/1(is_KeyPoint) -> is_Keypoint/1
  valid_in/1 -> detect_keypoint/4(valid_in), dog_space/5(valid_in), scale_space/2(valid_in)
  scale_space/2(scale3) -> dog_space/2(scale3_in)
  dog_space/1(dog3_out) -> detect_keypoint/1(pixel_dog3_in)
  dog_space/3(dog1_out) -> detect_keypoint/3(pixel_dog1_in)
  dog_space/2(dog2_out) -> detect_keypoint/2(pixel_dog2_in)
  data_in/1 -> scale_space/1(data_in)

== system twoOctave/sift/hist_bin/Bus_Concatenation ==
  orien : Inport
  bin1_in : Inport  Port=2
  bin2_in : Inport  Port=3
  biin3_in : Inport  Port=4
  bin4_in : Inport  Port=5
  bin5_in : Inport  Port=6
  bin6_in : Inport  Port=7
  bin_in : Inport  Port=8
  bin8_in : Inport  Port=9
  clken : Inport  Port=10
  Bus Concatenation{,1..3} (4 alike) : allblocks_alteradspbuilder2/Bus Concatenation  isSigned=off  awidth=16  bwidth=16  pipeline_display=0
  Bus Concatenation7 : allblocks_alteradspbuilder2/Bus Concatenation  isSigned=off  awidth=32  bwidth=32  pipeline_display=0
  Bus Concatenation8 : allblocks_alteradspbuilder2/Bus Concatenation  isSigned=off  awidth=32  bwidth=32  pipeline_display=0
  Bus Concatenation9 : allblocks_alteradspbuilder2/Bus Concatenation  isSigned=off  awidth=64  bwidth=64  pipeline_display=0
  Delay : allblocks_alteradspbuilder2/Delay  pipeline=1  pipeline_display=1  ClockPhase=1  use_ena=on  use_sclr=off  allowFloatingPointOverride=on  logOutputs=off  logFile=C:\Users\ASUS\Desktop\final_sift_fpga\tb_twoOctave\twoOctave_sift_hist%5Fbin_Bus%5FConcatenation_Delay.fixedpointlog  use_init=off  reset_value=1
  Multiplexer : allblocks_alteradspbuilder2/Multiplexer  numInputs=8  pipeline=1  oneHot=off  pipeline_display=1  use_ena=on  use_aclr=off  allowFloatingPointOverride=on  logOutputs=off  logFile=C:\Users\ASUS\Desktop\final_sift_fpga\tb_twoOctave\twoOctave_sift_hist%5Fbin_Bus%5FConcatenation_Multiplexer.fixedpointlog
  Multiplexer1 : allblocks_alteradspbuilder2/Multiplexer  numInputs=8  pipeline=1  oneHot=off  pipeline_display=1  use_ena=on  use_aclr=off  allowFloatingPointOverride=on  logOutputs=off  logFile=C:\Users\ASUS\Desktop\final_sift_fpga\tb_twoOctave\twoOctave_sift_hist%5Fbin_Bus%5FConcatenation_Multiplexer1.fixedpointlog
  Multiplexer2 : allblocks_alteradspbuilder2/Multiplexer  numInputs=8  pipeline=1  oneHot=off  pipeline_display=1  use_ena=on  use_aclr=off  allowFloatingPointOverride=on  logOutputs=off  logFile=C:\Users\ASUS\Desktop\final_sift_fpga\tb_twoOctave\twoOctave_sift_hist%5Fbin_Bus%5FConcatenation_Multiplexer2.fixedpointlog
  Multiplexer3 : allblocks_alteradspbuilder2/Multiplexer  numInputs=8  pipeline=1  oneHot=off  pipeline_display=1  use_ena=on  use_aclr=off  allowFloatingPointOverride=on  logOutputs=off  logFile=C:\Users\ASUS\Desktop\final_sift_fpga\tb_twoOctave\twoOctave_sift_hist%5Fbin_Bus%5FConcatenation_Multiplexer3.fixedpointlog
  Multiplexer4 : allblocks_alteradspbuilder2/Multiplexer  numInputs=8  pipeline=1  oneHot=off  pipeline_display=1  use_ena=on  use_aclr=off  allowFloatingPointOverride=on  logOutputs=off  logFile=C:\Users\ASUS\Desktop\final_sift_fpga\tb_twoOctave\twoOctave_sift_hist%5Fbin_Bus%5FConcatenation_Multiplexer4.fixedpointlog
  Multiplexer5 : allblocks_alteradspbuilder2/Multiplexer  numInputs=8  pipeline=1  oneHot=off  pipeline_display=1  use_ena=on  use_aclr=off  allowFloatingPointOverride=on  logOutputs=off  logFile=C:\Users\ASUS\Desktop\final_sift_fpga\tb_twoOctave\twoOctave_sift_hist%5Fbin_Bus%5FConcatenation_Multiplexer5.fixedpointlog
  Multiplexer6 : allblocks_alteradspbuilder2/Multiplexer  numInputs=8  pipeline=1  oneHot=off  pipeline_display=1  use_ena=on  use_aclr=off  allowFloatingPointOverride=on  logOutputs=off  logFile=C:\Users\ASUS\Desktop\final_sift_fpga\tb_twoOctave\twoOctave_sift_hist%5Fbin_Bus%5FConcatenation_Multiplexer6.fixedpointlog
  Multiplexer7 : allblocks_alteradspbuilder2/Multiplexer  numInputs=8  pipeline=1  oneHot=off  pipeline_display=1  use_ena=on  use_aclr=off  allowFloatingPointOverride=on  logOutputs=off  logFile=C:\Users\ASUS\Desktop\final_sift_fpga\tb_twoOctave\twoOctave_sift_hist%5Fbin_Bus%5FConcatenation_Multiplexer7.fixedpointlog
  To Workspace : ToWorkspace  VariableName=o1  SaveFormat=Timeseries  SampleTime=-1
  hist_bin : Outport
  Orien_out : Outport  Port=2
  wires:
  bin1_in/1 -> [bin1]
  bin2_in/1 -> [bin2]
  biin3_in/1 -> [bin3]
  bin4_in/1 -> [bin4]
  bin5_in/1 -> [bin5]
  bin6_in/1 -> [bin6]
  bin_in/1 -> [bin7]
  bin8_in/1 -> [bin8]
  Bus Concatenation/1 -> Bus Concatenation8/2
  [bin6_final] -> Bus Concatenation1/2
  Bus Concatenation1/1 -> Bus Concatenation8/1
  [bin8_final] -> Bus Concatenation/2
  [bin5_final] -> Bus Concatenation1/1
  [bin7_final] -> Bus Concatenation/1
  [bin4_final] -> Bus Concatenation2/2
  [bin3_final] -> Bus Concatenation2/1
  [bin2_final] -> Bus Concatenation3/2
  [bin1_final] -> Bus Concatenation3/1
  Bus Concatenation3/1 -> Bus Concatenation7/1
  Bus Concatenation2/1 -> Bus Concatenation7/2
  Bus Concatenation7/1 -> Bus Concatenation9/1
  Bus Concatenation8/1 -> Bus Concatenation9/2
  orien/1 -> [orien]
  clken/1 -> [clken]
  [bin1] -> Multiplexer/2
  [orien] -> Multiplexer/1
  [bin2] -> Multiplexer/3
  [bin3] -> Multiplexer/4
  [bin4] -> Multiplexer/5
  [bin5] -> Multiplexer/6
  [bin6] -> Multiplexer/7
  [bin7] -> Multiplexer/8
  [bin8] -> Multiplexer/9
  Multiplexer/1 -> [bin1_final]
  [clken] -> Multiplexer/10
  [bin2] -> Multiplexer1/2
  [orien] -> Multiplexer1/1
  [bin3] -> Multiplexer1/3
  [bin4] -> Multiplexer1/4
  [bin5] -> Multiplexer1/5
  [bin6] -> Multiplexer1/6
  [bin7] -> Multiplexer1/7
  [bin8] -> Multiplexer1/8
  [bin1] -> Multiplexer1/9
  Multiplexer1/1 -> [bin2_final]
  [clken] -> Multiplexer1/10
  [bin3] -> Multiplexer2/2
  [orien] -> Multiplexer2/1
  [bin4] -> Multiplexer2/3
  [bin5] -> Multiplexer2/4
  [bin6] -> Multiplexer2/5
  [bin7] -> Multiplexer2/6
  [bin8] -> Multiplexer2/7
  [bin1] -> Multiplexer2/8
  [bin2] -> Multiplexer2/9
  Multiplexer2/1 -> [bin3_final]
  [clken] -> Multiplexer2/10
  [bin4] -> Multiplexer3/2
  [orien] -> Multiplexer3/1
  [bin5] -> Multiplexer3/3
  [bin6] -> Multiplexer3/4
  [bin7] -> Multiplexer3/5
  [bin8] -> Multiplexer3/6
  [bin1] -> Multiplexer3/7
  [bin2] -> Multiplexer3/8
  [bin3] -> Multiplexer3/9
  Multiplexer3/1 -> [bin4_final]
  [clken] -> Multiplexer3/10
  [bin5] -> Multiplexer4/2
  [orien] -> Multiplexer4/1
  [bin6] -> Multiplexer4/3
  [bin7] -> Multiplexer4/4
  [bin8] -> Multiplexer4/5
  [bin1] -> Multiplexer4/6
  [bin2] -> Multiplexer4/7
  [bin3] -> Multiplexer4/8
  [bin4] -> Multiplexer4/9
  Multiplexer4/1 -> [bin5_final]
  [clken] -> Multiplexer4/10
  [bin6] -> Multiplexer5/2
  [orien] -> Multiplexer5/1
  [bin7] -> Multiplexer5/3
  [bin8] -> Multiplexer5/4
  [bin1] -> Multiplexer5/5
  [bin2] -> Multiplexer5/6
  [bin3] -> Multiplexer5/7
  [bin4] -> Multiplexer5/8
  [bin5] -> Multiplexer5/9
  Multiplexer5/1 -> [bin6_final]
  [clken] -> Multiplexer5/10
  [bin7] -> Multiplexer6/2
  [orien] -> Multiplexer6/1
  [bin8] -> Multiplexer6/3
  [bin1] -> Multiplexer6/4
  [bin2] -> Multiplexer6/5
  [bin3] -> Multiplexer6/6
  [bin4] -> Multiplexer6/7
  [bin5] -> Multiplexer6/8
  [bin6] -> Multiplexer6/9
  Multiplexer6/1 -> [bin7_final]
  [clken] -> Multiplexer6/10
  [bin8] -> Multiplexer7/2
  [orien] -> Multiplexer7/1
  [bin1] -> Multiplexer7/3
  [bin2] -> Multiplexer7/4
  [bin3] -> Multiplexer7/5
  [bin4] -> Multiplexer7/6
  [bin5] -> Multiplexer7/7
  [bin6] -> Multiplexer7/8
  [bin7] -> Multiplexer7/9
  Multiplexer7/1 -> [bin8_final]
  [clken] -> Multiplexer7/10
  Bus Concatenation9/1 -> hist_bin/1
  [orien] -> Delay/1
  Delay/1 -> Orien_out/1, To Workspace/1
  [clken] -> Delay/2
